simulink model "motorModel"  (R2017a)
settings: Solver=VariableStepAuto  StartTime=0.0  StopTime=1  RelTol=1e-3
settings Model: Creator=root  LastModifiedBy=root

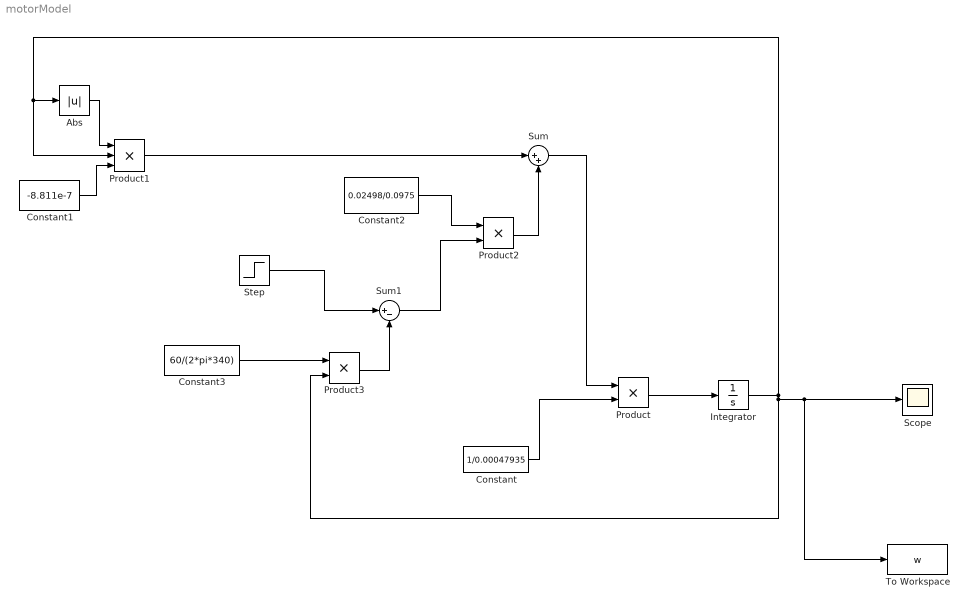
== system motorModel ==
  Abs : Abs
  Constant : Constant  Value=1/0.00047935
  Constant1 : Constant  Value=-8.811e-7
  Constant2 : Constant  Value=0.02498/0.0975
  Constant3 : Constant  Value=60/(2*pi*340)
  Integrator : Integrator
  Product : Product
  Product1 : Product  Inputs=3
  Product2 : Product
  Product3 : Product
  Scope : Scope
  Step : Step  Time=0  After=2.2  SampleTime=0
  Sum : Sum  Inputs=|++
  Sum1 : Sum  Inputs=|+-
  To Workspace : ToWorkspace  VariableName=w  SaveFormat=Timeseries  SampleTime=-1
  wires:
  Product/1 -> Integrator/1
  Constant/1 -> Product/2
  Integrator/1 -> To Workspace/1, Scope/1, Product3/2, Product1/2, Abs/1
  Abs/1 -> Product1/1
  Constant1/1 -> Product1/3
  Sum/1 -> Product/1
  Product1/1 -> Sum/1
  Product2/1 -> Sum/2
  Constant2/1 -> Product2/1
  Sum1/1 -> Product2/2
  Step/1 -> Sum1/1
  Product3/1 -> Sum1/2
  Constant3/1 -> Product3/1
